simulink model "envelope_2"  (R2017a)
settings: Solver=VariableStepAuto  StartTime=0.0  StopTime=10.0  RelTol=1e-3
settings Model: Creator=Andre  LastModifiedBy=Andre

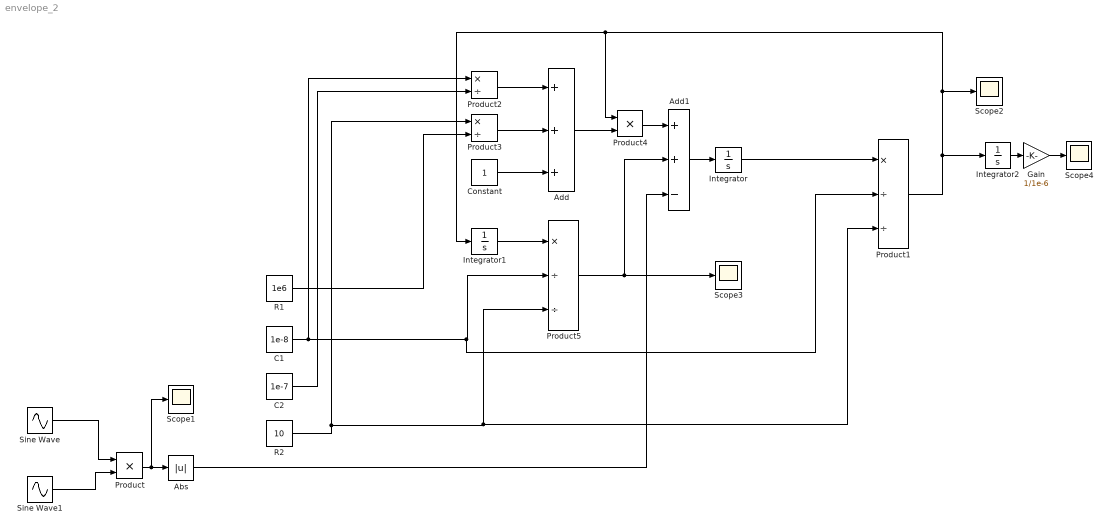
== system envelope_2 ==
  Abs : Abs
  Add : Sum  Inputs=+++
  Add1 : Sum  Inputs=++-
  "C1 " : Constant  Value=1e-8
  C2 : Constant  Value=1e-7
  Constant : Constant
  Gain : Gain  Gain=1/1e-6
  Integrator : Integrator
  Integrator1 : Integrator
  Integrator2 : Integrator
  Product : Product
  Product1 : Product  Inputs=*//
  Product2 : Product  Inputs=*/
  Product3 : Product  Inputs=*/
  Product4 : Product
  Product5 : Product  Inputs=*//
  R1 : Constant  Value=1e6
  R2 : Constant  Value=10
  Scope{1..4} (4 alike) : Scope
  Sine Wave : Sin  Frequency=100  SampleTime=0
  Sine Wave1 : Sin  SampleTime=0
  wires:
  Product/1 -> Scope1/1, Abs/1
  Sine Wave1/1 -> Product/2
  Sine Wave/1 -> Product/1
  C2/1 -> Product2/2
  R2/1 -> Product3/1, Product1/3, Product5/3
  Integrator/1 -> Product1/1
  Constant/1 -> Add/3
  Product3/1 -> Add/2
  Product2/1 -> Add/1
  Add/1 -> Product4/2
  Product4/1 -> Add1/1
  Add1/1 -> Integrator/1
  Integrator1/1 -> Product5/1
  Product5/1 -> Scope3/1, Add1/2
  Abs/1 -> Add1/3
  "C1 "/1 -> Product2/1, Product1/2, Product5/2
  R1/1 -> Product3/2
  Product1/1 -> Integrator2/1, Scope2/1, Integrator1/1, Product4/1
  Integrator2/1 -> Gain/1
  Gain/1 -> Scope4/1
